simulink model "q_2dsfl_pos_cntrl"  (Simulink 7.0)
settings: Solver=ode1  StartTime=0.0  StopTime=inf  FixedStep=0.002  RelTol=1e-3
undefined symbols (not defined in the file or in its folder): DTH1_LIM_ENABLE, DTH2_LIM_ENABLE, DTH2_MAX, DTH2_MIN, HIL, K1, K1_defl_b, K1_strain_b, K2, K2_defl_b, K2_strain_b, KE_D1, KE_D2, LIMIT_SWITCHES_ENABLE, qc_get_step_size, wcf, wcfa, zetaf
libraries: quarc_library x21, simulink_extras x8, simulink x6
settings Model: Creator=ajavid  LastModifiedBy=MLevis  SimulationMode=external  ExtModeTrigDuration=60000
settings SolverCC: PositivePriorityOrder=on
settings DataIOCC: MaxDataPoints=30000
settings DebuggingCC: SaveWithParameterizedLinksMsg=none
settings RTWCC: SystemTargetFile=quarc_windows.tlc  TemplateMakefile=quarc_default_tmf  Description=QuaRC Win32 Target  ProcessScript=quarc_windows_make_rtw_hook
settings STFCustomTargetCC: TargetFcnLib=ansi_tfl_tmw.mat  TargetPreCompLibLocation=C:\DOCUME~1\ALLUSE~1\APPLIC~1\QUARC\lib\2007b\windows\release  GenFloatMathFcnCalls=ANSI_C  SystemTargetFile=quarc_windows.tlc
settings GRTTargetCC: TargetFcnLib=ansi_tfl_tmw.mat  TargetPreCompLibLocation=C:\DOCUME~1\ALLUSE~1\APPLIC~1\QUARC\lib\2007b\windows\release  CompOptLevelCompliant=off  MatFileLogging=off  ExtMode=on  ExtModeMexFile=quarc_comm

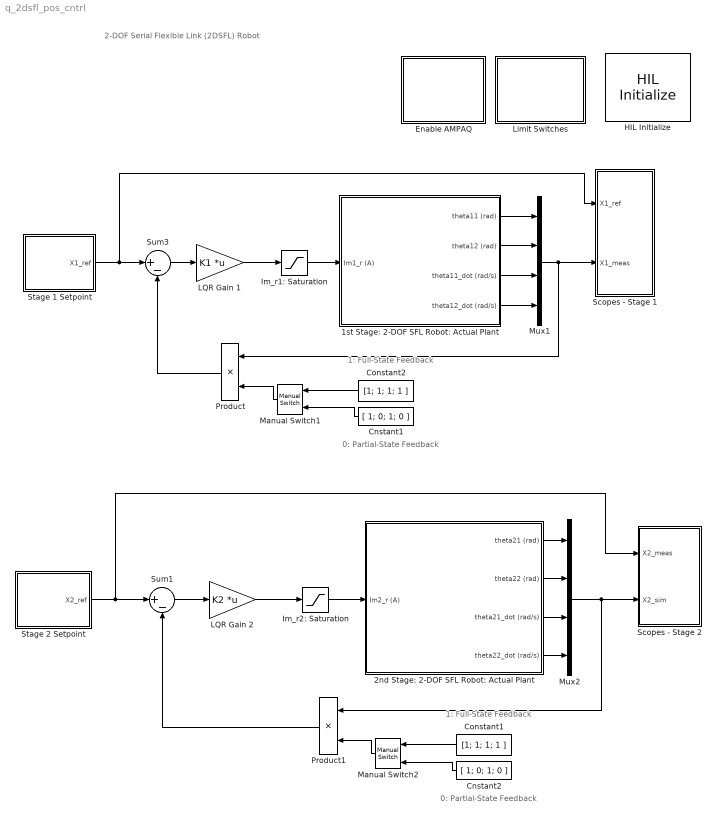
== system q_2dsfl_pos_cntrl ==
  note: 2-DOF Serial Flexible Link (2DSFL) Robot
  note: 1: Full-State Feedback
  note: 0: Partial-State Feedback
  note: 1: Full-State Feedback
  note: 0: Partial-State Feedback
  1st Stage: 2-DOF SFL Robot: Actual Plant : Subsystem
  2nd Stage: 2-DOF SFL Robot: Actual Plant : Subsystem
  Cnstant1 : Constant  Orientation=left  Value=[ 1; 0; 1; 0 ]  OutDataType=sfix(16)  OutScaling=2^0
  Cnstant2 : Constant  Orientation=left  Value=[ 1; 0; 1; 0 ]  OutDataType=sfix(16)  OutScaling=2^0
  Constant1 : Constant  Orientation=left  Value=[1; 1; 1; 1 ]  OutDataType=sfix(16)  OutScaling=2^0
  Constant2 : Constant  Orientation=left  Value=[1; 1; 1; 1 ]  OutDataType=sfix(16)  OutScaling=2^0
  Enable AMPAQ : Subsystem
  HIL Initialize : quarc_library/Data Acquisition/Generic/Configuration/HIL Initialize  object_name=HIL-1  board_type=q8  board_number=0  exclusive=off  active=on  hardware_clocks=[0:1]  clock_modes=[0 0]  initial_clock_frequencies=[]  set_clock_params_at_start=on  set_clock_params_at_switch_in=off  set_clock_frequencies_at_start=off  set_clock_frequencies_at_switch_in=off  analog_input_channels=[0:7]  analog_input_maximums=10  analog_input_minimums=-10  set_analog_input_params_at_start=off  set_analog_input_params_at_switch_in=off  analog_output_channels=[0:7]  analog_output_maximums=[10]  analog_output_minimums=[-10]  initial_analog_outputs=[0]  final_analog_outputs=[0]  watchdog_analog_outputs=0  set_analog_output_params_at_start=on  set_analog_output_params_at_switch_in=off  set_analog_outputs_at_start=on  set_analog_outputs_at_switch_in=off  set_analog_outputs_at_terminate=on  set_analog_outputs_at_switch_out=off  set_analog_outputs_on_watchdog=off  digital_input_channels=[8:31]  digital_output_channels=[0:7]  digital_output_configuration=[]  initial_digital_outputs=[1]  final_digital_outputs=[1]  watchdog_digital_outputs=[2]  set_digital_output_params_at_start=off  set_digital_output_params_at_switch_in=off  set_digital_outputs_at_start=on  set_digital_outputs_at_switch_in=off  set_digital_outputs_at_terminate=on  set_digital_outputs_at_switch_out=off  set_digital_outputs_on_watchdog=on  encoder_channels=[0:7]  quadrature=[4]  encoder_filter_frequency=(1/120e-9)/1  initial_encoder_counts=[0]  set_encoder_params_at_start=on  set_encoder_params_at_switch_in=off  set_encoder_counts_at_start=on  set_encoder_counts_at_switch_in=off  pwm_channels=[]  pwm_modes=[0]  pwm_frequency=(1/60e-9)/1024  pwm_configuration=[]  pwm_alignment=[]  pwm_polarity=[]  pwm_leading_deadband=[]  pwm_trailing_deadband=[]  initial_pwm_outputs=[0]  final_pwm_outputs=[0]  watchdog_pwm_outputs=[]  set_pwm_params_at_start=on  set_pwm_params_at_switch_in=off  set_pwm_outputs_at_start=on  set_pwm_outputs_at_switch_in=off  set_pwm_outputs_at_terminate=on  set_pwm_outputs_at_switch_out=off  set_pwm_outputs_on_watchdog=off  other_output_channels=[]  initial_other_outputs=[]  final_other_outputs=[]  watchdog_other_outputs=[]  set_other_outputs_at_start=off  set_other_outputs_at_switch_in=off  set_other_outputs_at_terminate=off  set_other_outputs_at_switch_out=off  set_other_outputs_on_watchdog=off
  Im_r1: Saturation : Saturate  UpperLimit=0.94  LowerLimit=-0.94
  Im_r2: Saturation : Saturate  UpperLimit=1.2  LowerLimit=-1.2
  LQR Gain 1 : Gain  Gain=K1  Multiplication=Matrix(K*u)  ParameterDataType=sfix(16)  ParameterScaling=2^0  OutDataType=sfix(16)  OutScaling=2^0
  LQR Gain 2 : Gain  Gain=K2  Multiplication=Matrix(K*u)  ParameterDataType=sfix(16)  ParameterScaling=2^0  OutDataType=sfix(16)  OutScaling=2^0
  Limit Switches : Subsystem
  Manual Switch1 : simulink/Signal Routing/Manual Switch  Orientation=left  SystemSampleTime=-1  sw=1  action=0  varsize=off
  Manual Switch2 : simulink/Signal Routing/Manual Switch  Orientation=left  SystemSampleTime=-1  sw=1  action=0  varsize=off
  Mux1 : Mux
  Mux2 : Mux
  Product : Product  Orientation=left  OutDataType=sfix(16)  OutScaling=2^0  SaturateOnIntegerOverflow=on  RndMeth=Zero  InputSameDT=on
  Product1 : Product  Orientation=left  OutDataType=sfix(16)  OutScaling=2^0  SaturateOnIntegerOverflow=on  RndMeth=Zero  InputSameDT=on
  Scopes - Stage 1 : Subsystem
  Scopes - Stage 2 : Subsystem
  Stage 1 Setpoint : Subsystem
  Stage 2 Setpoint : Subsystem
  Sum1 : Sum  Inputs=|+-  OutDataType=sfix(16)  OutScaling=2^0  SaturateOnIntegerOverflow=on  InputSameDT=on
  Sum3 : Sum  Inputs=|+-  OutDataType=sfix(16)  OutScaling=2^0  SaturateOnIntegerOverflow=on  InputSameDT=on
  wires:
  1st Stage: 2-DOF SFL Robot: Actual Plant/3(theta11_dot (rad/s)) -> Mux1/3
  1st Stage: 2-DOF SFL Robot: Actual Plant/4(theta12_dot (rad/s)) -> Mux1/4
  1st Stage: 2-DOF SFL Robot: Actual Plant/2(theta12 (rad)) -> Mux1/2
  1st Stage: 2-DOF SFL Robot: Actual Plant/1(theta11 (rad)) -> Mux1/1
  Mux1/1 -> Product/1, Scopes - Stage 1/2(X1_meas)
  2nd Stage: 2-DOF SFL Robot: Actual Plant/3(theta21_dot (rad/s)) -> Mux2/3
  2nd Stage: 2-DOF SFL Robot: Actual Plant/4(theta22_dot (rad/s)) -> Mux2/4
  2nd Stage: 2-DOF SFL Robot: Actual Plant/2(theta22 (rad)) -> Mux2/2
  2nd Stage: 2-DOF SFL Robot: Actual Plant/1(theta21 (rad)) -> Mux2/1
  Im_r2: Saturation/1 -> 2nd Stage: 2-DOF SFL Robot: Actual Plant/1(Im2_r (A))
  Constant2/1 -> Manual Switch1/1
  Cnstant1/1 -> Manual Switch1/2
  Manual Switch1/1 -> Product/2
  Im_r1: Saturation/1 -> 1st Stage: 2-DOF SFL Robot: Actual Plant/1(Im1_r (A))
  Stage 1 Setpoint/1(X1_ref) -> Sum3/1, Scopes - Stage 1/1(X1_ref)
  Sum3/1 -> LQR Gain 1/1
  Product/1 -> Sum3/2
  Stage 2 Setpoint/1(X2_ref) -> Sum1/1, Scopes - Stage 2/1(X2_meas)
  Sum1/1 -> LQR Gain 2/1
  LQR Gain 2/1 -> Im_r2: Saturation/1
  Mux2/1 -> Scopes - Stage 2/2(X2_sim), Product1/1
  LQR Gain 1/1 -> Im_r1: Saturation/1
  Constant1/1 -> Manual Switch2/1
  Cnstant2/1 -> Manual Switch2/2
  Manual Switch2/1 -> Product1/2
  Product1/1 -> Sum1/2

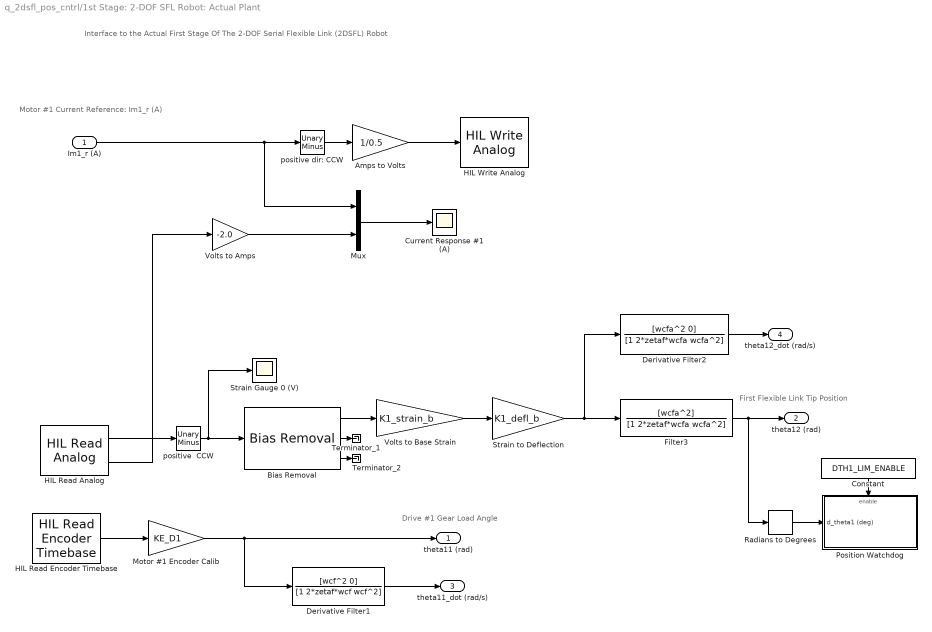
== system q_2dsfl_pos_cntrl/1st Stage: 2-DOF SFL Robot: Actual Plant ==
  note: Interface to the Actual
      | First Stage Of The 2-DOF Serial Flexible Link (2DSFL) Robot
  note: First Flexible Link
      | Tip Position
  note: Drive #1
      | Gear Load Angle
  note: Motor #1 Current Reference:
      | Im1_r (A)
  Im1_r (A) : Inport  OutDataType=sfix(16)  OutScaling=2^0
  Amps to Volts : Gain  Gain=1/0.5  ParameterDataType=sfix(16)  ParameterScaling=2^0  OutDataType=sfix(16)  OutScaling=2^0  SaturateOnIntegerOverflow=on
  Bias Removal : quarc_library/Discrete/Bias Removal  SystemSampleTime=-1  start_time=0  end_time=1  switch_id=0  sample_time=qc_get_step_size
  Constant : Constant  Orientation=down  Value=DTH1_LIM_ENABLE  OutDataType=sfix(16)  OutScaling=2^0
  Current Response #1 (A) : Scope
      settings: TimeRange=20  YMin=-1  YMax=1  SaveName=data_Im1  DataFormat=Array  MaxDataPoints=10000
  Derivative Filter1 : TransferFcn  Numerator=[wcf^2 0]  Denominator=[1 2*zetaf*wcf wcf^2]
  Derivative Filter2 : TransferFcn  Numerator=[wcfa^2 0]  Denominator=[1 2*zetaf*wcfa wcfa^2]
  Filter3 : TransferFcn  Numerator=[wcfa^2]  Denominator=[1 2*zetaf*wcfa wcfa^2]
  HIL Read Analog : quarc_library/Data Acquisition/Generic/Immediate I//O/HIL Read Analog  object_name=HIL-1  channels=[0,2]  sample_time=qc_get_step_size  active=on  vector_output=off
  HIL Read Encoder Timebase : quarc_library/Data Acquisition/Generic/Timebases/HIL Read Encoder Timebase  object_name=HIL-1  clock=0  channels=0  samples_in_buffer=max(ceil(1/qc_get_step_size), 1)  active=on  vector_output=off  data_type_mode=Inherit via back propagation  data_type=double
  HIL Write Analog : quarc_library/Data Acquisition/Generic/Immediate I//O/HIL Write Analog  object_name=HIL-1  channels=0  sample_time=-1  active=off  vector_input=off
  Motor #1 Encoder Calib : Gain  Gain=KE_D1  ParameterDataType=sfix(16)  ParameterScaling=2^0  OutDataType=sfix(16)  OutScaling=2^0  SaturateOnIntegerOverflow=on
  Mux : Mux  Inputs=2
  Position Watchdog : Subsystem  TreatAsAtomicUnit=on
  Radians to Degrees : simulink_extras/Transformations/Radians to Degrees  SystemSampleTime=-1
  Strain Gauge 0 (V) : Scope
      settings: TickLabels=on  TimeRange=2  YMin=-1.5  YMax=1.5  SaveName=ScopeData7  DataFormat=Array
  Strain to Deflection : Gain  Gain=K1_defl_b  ParameterDataType=sfix(16)  ParameterScaling=2^0  OutDataType=sfix(16)  OutScaling=2^0  SaturateOnIntegerOverflow=on
  Terminator_1 : Terminator
  Terminator_2 : Terminator
  Volts to Amps : Gain  Gain=-2.0  ParameterDataType=sfix(16)  ParameterScaling=2^0  OutDataType=sfix(16)  OutScaling=2^0
  Volts to Base Strain : Gain  Gain=K1_strain_b  ParameterDataType=sfix(16)  ParameterScaling=2^0  OutDataType=sfix(16)  OutScaling=2^0  SaturateOnIntegerOverflow=on
  positive  CCW : simulink/Math Operations/Unary Minus  DoSatur=off
  positive dir: CCW : simulink/Math Operations/Unary Minus  DoSatur=off
  theta11 (rad) : Outport  OutDataType=sfix(16)  OutScaling=2^0  InitialOutput=0
  theta12 (rad) : Outport  Port=2  OutDataType=sfix(16)  OutScaling=2^0  InitialOutput=0
  theta11_dot (rad/s) : Outport  Port=3  OutDataType=sfix(16)  OutScaling=2^0  InitialOutput=0
  theta12_dot (rad/s) : Outport  Port=4  OutDataType=sfix(16)  OutScaling=2^0  InitialOutput=0
  wires:
  positive  CCW/1 -> Strain Gauge 0 (V)/1, Bias Removal/1
  Filter3/1 -> theta12 (rad)/1, Radians to Degrees/1
  Derivative Filter1/1 -> theta11_dot (rad/s)/1
  Derivative Filter2/1 -> theta12_dot (rad/s)/1
  Strain to Deflection/1 -> Filter3/1, Derivative Filter2/1
  Im1_r (A)/1 -> positive dir: CCW/1, Mux/1
  HIL Read Encoder Timebase/1 -> Motor #1 Encoder Calib/1
  Volts to Amps/1 -> Mux/2
  Mux/1 -> Current Response #1 (A)/1
  Motor #1 Encoder Calib/1 -> Derivative Filter1/1, theta11 (rad)/1
  HIL Read Analog/1 -> positive  CCW/1
  positive dir: CCW/1 -> Amps to Volts/1
  Volts to Base Strain/1 -> Strain to Deflection/1
  Amps to Volts/1 -> HIL Write Analog/1
  HIL Read Analog/2 -> Volts to Amps/1
  Constant/1 -> Position Watchdog/Enable
  Radians to Degrees/1 -> Position Watchdog/1(d_theta1 (deg))
  Bias Removal/1 -> Volts to Base Strain/1
  Bias Removal/2 -> Terminator_1/1
  Bias Removal/3 -> Terminator_2/1

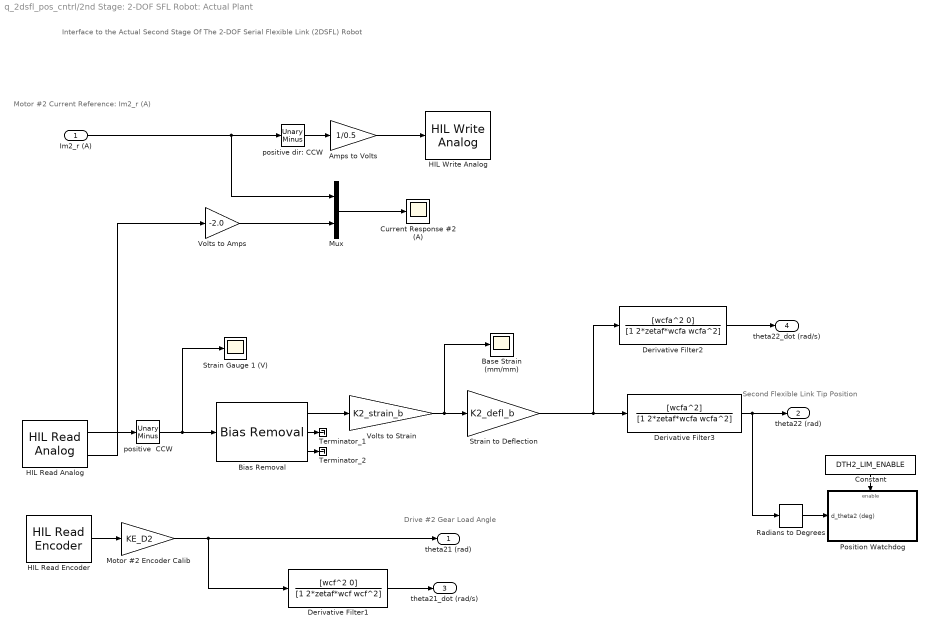
== system q_2dsfl_pos_cntrl/2nd Stage: 2-DOF SFL Robot: Actual Plant ==
  note: Motor #2 Current Reference:
      | Im2_r (A)
  note: Drive #2
      | Gear Load Angle
  note: Second Flexible Link
      | Tip Position
  note: Interface to the Actual
      | Second Stage Of The 2-DOF Serial Flexible Link (2DSFL) Robot
  Im2_r (A) : Inport  OutDataType=sfix(16)  OutScaling=2^0
  Amps to Volts : Gain  Gain=1/0.5  ParameterDataType=sfix(16)  ParameterScaling=2^0  OutDataType=sfix(16)  OutScaling=2^0  SaturateOnIntegerOverflow=on
  Base Strain (mm/mm) : Scope
      settings: TickLabels=on  TimeRange=1.000000  YMin=-1  YMax=1  SaveName=ScopeData4  DataFormat=Array
  Bias Removal : quarc_library/Discrete/Bias Removal  SystemSampleTime=-1  start_time=0  end_time=0.2  switch_id=0  sample_time=qc_get_step_size
  Constant : Constant  Orientation=down  Value=DTH2_LIM_ENABLE  OutDataType=sfix(16)  OutScaling=2^0
  Current Response #2 (A) : Scope
      settings: TimeRange=20  YMin=-1.25  YMax=1.25  SaveName=data_Im2  DataFormat=Array  MaxDataPoints=10000
  Derivative Filter1 : TransferFcn  Numerator=[wcf^2 0]  Denominator=[1 2*zetaf*wcf wcf^2]
  Derivative Filter2 : TransferFcn  Numerator=[wcfa^2 0]  Denominator=[1 2*zetaf*wcfa wcfa^2]
  Derivative Filter3 : TransferFcn  Numerator=[wcfa^2]  Denominator=[1 2*zetaf*wcfa wcfa^2]
  HIL Read Analog : quarc_library/Data Acquisition/Generic/Immediate I//O/HIL Read Analog  object_name=HIL-1  channels=[1,3]  sample_time=qc_get_step_size  active=on  vector_output=off
  HIL Read Encoder : quarc_library/Data Acquisition/Generic/Immediate I//O/HIL Read Encoder  object_name=HIL-1  channels=1  sample_time=qc_get_step_size  active=on  vector_output=off  data_type_mode=Inherit via back propagation  data_type=double
  HIL Write Analog : quarc_library/Data Acquisition/Generic/Immediate I//O/HIL Write Analog  object_name=HIL-1  channels=1  sample_time=-1  active=off  vector_input=off
  Motor #2 Encoder Calib : Gain  Gain=KE_D2  ParameterDataType=sfix(16)  ParameterScaling=2^0  OutDataType=sfix(16)  OutScaling=2^0  SaturateOnIntegerOverflow=on
  Mux : Mux  Inputs=2
  Position Watchdog : Subsystem  TreatAsAtomicUnit=on
  Radians to Degrees : simulink_extras/Transformations/Radians to Degrees  SystemSampleTime=-1
  Strain Gauge 1 (V) : Scope
      settings: TickLabels=on  TimeRange=1.000000  YMin=-1  YMax=1  SaveName=ScopeData7  DataFormat=Array
  Strain to Deflection : Gain  Gain=K2_defl_b  ParameterDataType=sfix(16)  ParameterScaling=2^0  OutDataType=sfix(16)  OutScaling=2^0  SaturateOnIntegerOverflow=on
  Terminator_1 : Terminator
  Terminator_2 : Terminator
  Volts to Amps : Gain  Gain=-2.0  ParameterDataType=sfix(16)  ParameterScaling=2^0  OutDataType=sfix(16)  OutScaling=2^0
  Volts to Strain : Gain  Gain=K2_strain_b  ParameterDataType=sfix(16)  ParameterScaling=2^0  OutDataType=sfix(16)  OutScaling=2^0  SaturateOnIntegerOverflow=on
  positive  CCW : simulink/Math Operations/Unary Minus  DoSatur=off
  positive dir: CCW : simulink/Math Operations/Unary Minus  DoSatur=off
  theta21 (rad) : Outport  OutDataType=sfix(16)  OutScaling=2^0  InitialOutput=0
  theta22 (rad) : Outport  Port=2  OutDataType=sfix(16)  OutScaling=2^0  InitialOutput=0
  theta21_dot (rad/s) : Outport  Port=3  OutDataType=sfix(16)  OutScaling=2^0  InitialOutput=0
  theta22_dot (rad/s) : Outport  Port=4  OutDataType=sfix(16)  OutScaling=2^0  InitialOutput=0
  wires:
  Derivative Filter3/1 -> theta22 (rad)/1, Radians to Degrees/1
  positive  CCW/1 -> Strain Gauge 1 (V)/1, Bias Removal/1
  Derivative Filter2/1 -> theta22_dot (rad/s)/1
  Strain to Deflection/1 -> Derivative Filter3/1, Derivative Filter2/1
  Derivative Filter1/1 -> theta21_dot (rad/s)/1
  Volts to Strain/1 -> Strain to Deflection/1, Base Strain (mm/mm)/1
  HIL Read Analog/1 -> positive  CCW/1
  HIL Read Analog/2 -> Volts to Amps/1
  Mux/1 -> Current Response #2 (A)/1
  Volts to Amps/1 -> Mux/2
  HIL Read Encoder/1 -> Motor #2 Encoder Calib/1
  Motor #2 Encoder Calib/1 -> theta21 (rad)/1, Derivative Filter1/1
  Im2_r (A)/1 -> positive dir: CCW/1, Mux/1
  Amps to Volts/1 -> HIL Write Analog/1
  Bias Removal/1 -> Volts to Strain/1
  Constant/1 -> Position Watchdog/Enable
  Radians to Degrees/1 -> Position Watchdog/1(d_theta2 (deg))
  Bias Removal/2 -> Terminator_1/1
  positive dir: CCW/1 -> Amps to Volts/1
  Bias Removal/3 -> Terminator_2/1

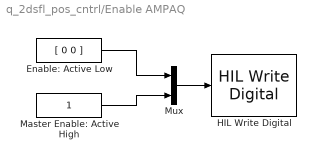
== system q_2dsfl_pos_cntrl/Enable AMPAQ ==
  Enable: Active Low : Constant  Value=[ 0 0 ]  OutDataType=sfix(16)  OutScaling=2^0
  HIL Write Digital : quarc_library/Data Acquisition/Generic/Immediate I//O/HIL Write Digital  object_name=HIL-1  channels=[0 1 4]  sample_time=-1  active=off  vector_input=on
  Master Enable: Active High : Constant  OutDataType=sfix(16)  OutScaling=2^0
  Mux : Mux  Inputs=2
  wires:
  Master Enable: Active High/1 -> Mux/2
  Enable: Active Low/1 -> Mux/1
  Mux/1 -> HIL Write Digital/1

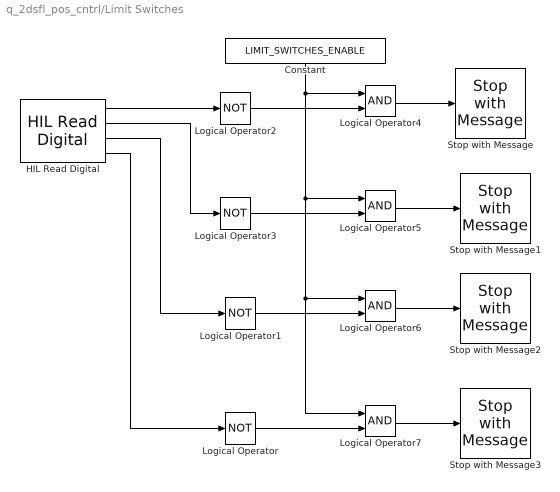
== system q_2dsfl_pos_cntrl/Limit Switches ==
  Constant : Constant  Orientation=down  Value=LIMIT_SWITCHES_ENABLE  OutDataType=sfix(16)  OutScaling=2^0
  HIL Read Digital : quarc_library/Data Acquisition/Generic/Immediate I//O/HIL Read Digital  object_name=HIL-1  channels=[8:11]  sample_time=qc_get_step_size  active=on  vector_output=off  data_type_mode=Inherit via back propagation  data_type=boolean
      settings: AttributesFormatString=(%<object_name>)
  Logical Operator{,1..3} (4 alike) : Logic  Operator=NOT  AllPortsSameDT=off  OutDataTypeMode=boolean
  Logical Operator{4..7} (4 alike) : Logic  AllPortsSameDT=off  OutDataTypeMode=boolean
  Stop with Message : quarc_library/Sinks/Error Handling/Stop with Message  SystemSampleTime=-1  message_type=Fixed error message  message_icon=Error  message=STAGE 1: MAX limit switch hit.
  Stop with Message1 : quarc_library/Sinks/Error Handling/Stop with Message  SystemSampleTime=-1  message_type=Fixed error message  message_icon=Error  message=STAGE 1: MIN limit switch hit.
  Stop with Message2 : quarc_library/Sinks/Error Handling/Stop with Message  SystemSampleTime=-1  message_type=Fixed error message  message_icon=Error  message=STAGE 2: MAX limit switch hit.
  Stop with Message3 : quarc_library/Sinks/Error Handling/Stop with Message  SystemSampleTime=-1  message_type=Fixed error message  message_icon=Error  message=STAGE 2: MIN limit switch hit.
  wires:
  Logical Operator7/1 -> Stop with Message3/1
  Logical Operator6/1 -> Stop with Message2/1
  Logical Operator5/1 -> Stop with Message1/1
  Logical Operator4/1 -> Stop with Message/1
  HIL Read Digital/4 -> Logical Operator/1
  HIL Read Digital/3 -> Logical Operator1/1
  HIL Read Digital/2 -> Logical Operator3/1
  HIL Read Digital/1 -> Logical Operator2/1
  Logical Operator2/1 -> Logical Operator4/2
  Constant/1 -> Logical Operator4/1, Logical Operator5/1, Logical Operator6/1, Logical Operator7/1
  Logical Operator3/1 -> Logical Operator5/2
  Logical Operator1/1 -> Logical Operator6/2
  Logical Operator/1 -> Logical Operator7/2

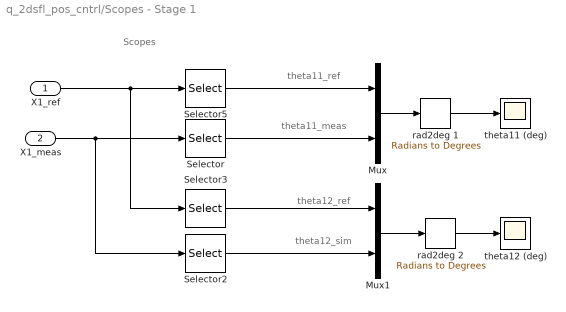
== system q_2dsfl_pos_cntrl/Scopes - Stage 1 ==
  note: Scopes
  note: theta12_sim
  note: theta11_ref
  note: theta11_meas
  note: theta12_ref
  X1_ref : Inport  OutDataType=sfix(16)  OutScaling=2^0
  X1_meas : Inport  Port=2  OutDataType=sfix(16)  OutScaling=2^0
  Mux : Mux  Inputs=2
  Mux1 : Mux  Inputs=2
  Selector : Selector  InputPortWidth=4  IndexOptions=Index vector (dialog)  Indices=[1]  OutputSizes=1
  Selector2 : Selector  InputPortWidth=4  IndexOptions=Index vector (dialog)  Indices=[2]  OutputSizes=1
  Selector3 : Selector  InputPortWidth=4  IndexOptions=Index vector (dialog)  Indices=[2]  OutputSizes=1
  Selector5 : Selector  InputPortWidth=4  IndexOptions=Index vector (dialog)  Indices=[1]  OutputSizes=1
  rad2deg 1 : simulink_extras/Transformations/Radians to Degrees  SystemSampleTime=-1
  rad2deg 2 : simulink_extras/Transformations/Radians to Degrees  SystemSampleTime=-1
  theta11 (deg) : Scope
      settings: TickLabels=on  TimeRange=20  YMin=-30  YMax=30  SaveName=data_th11  DataFormat=Array  MaxDataPoints=10000
  theta12 (deg) : Scope
      settings: TimeRange=20  YMin=-2  YMax=2  SaveName=data_th12  DataFormat=Array  MaxDataPoints=10000
  wires:
  X1_ref/1 -> Selector3/1, Selector5/1
  Mux/1 -> rad2deg 1/1
  Mux1/1 -> rad2deg 2/1
  X1_meas/1 -> Selector/1, Selector2/1
  rad2deg 1/1 -> theta11 (deg)/1
  rad2deg 2/1 -> theta12 (deg)/1
  Selector5/1 -> Mux/1
  Selector/1 -> Mux/2
  Selector2/1 -> Mux1/2
  Selector3/1 -> Mux1/1

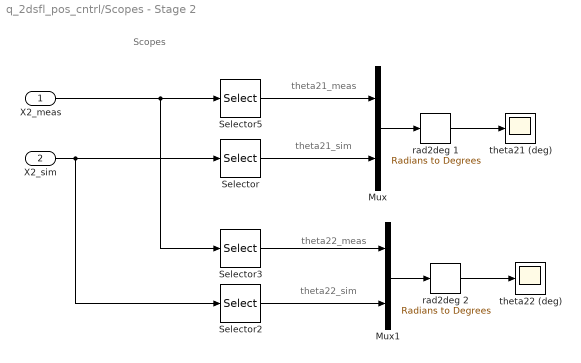
== system q_2dsfl_pos_cntrl/Scopes - Stage 2 ==
  note: Scopes
  note: theta22_sim
  note: theta21_sim
  note: theta21_meas
  note: theta22_meas
  X2_meas : Inport  OutDataType=sfix(16)  OutScaling=2^0
  X2_sim : Inport  Port=2  OutDataType=sfix(16)  OutScaling=2^0
  Mux : Mux  Inputs=2
  Mux1 : Mux  Inputs=2
  Selector : Selector  InputPortWidth=4  IndexOptions=Index vector (dialog)  Indices=[1]  OutputSizes=1
  Selector2 : Selector  InputPortWidth=4  IndexOptions=Index vector (dialog)  Indices=[2]  OutputSizes=1
  Selector3 : Selector  InputPortWidth=4  IndexOptions=Index vector (dialog)  Indices=[2]  OutputSizes=1
  Selector5 : Selector  InputPortWidth=4  IndexOptions=Index vector (dialog)  Indices=[1]  OutputSizes=1
  rad2deg 1 : simulink_extras/Transformations/Radians to Degrees  SystemSampleTime=-1
  rad2deg 2 : simulink_extras/Transformations/Radians to Degrees  SystemSampleTime=-1
  theta21 (deg) : Scope
      settings: TickLabels=on  TimeRange=20  YMin=-15  YMax=15  SaveName=data_th21  DataFormat=Array  MaxDataPoints=10000
  theta22 (deg) : Scope
      settings: TimeRange=20  YMin=-2.5  YMax=2.5  SaveName=data_th22  DataFormat=Array  MaxDataPoints=10000
  wires:
  Mux/1 -> rad2deg 1/1
  Mux1/1 -> rad2deg 2/1
  X2_meas/1 -> Selector3/1, Selector5/1
  X2_sim/1 -> Selector2/1, Selector/1
  rad2deg 1/1 -> theta21 (deg)/1
  rad2deg 2/1 -> theta22 (deg)/1
  Selector3/1 -> Mux1/1
  Selector2/1 -> Mux1/2
  Selector5/1 -> Mux/1
  Selector/1 -> Mux/2

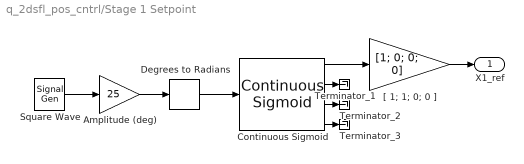
== system q_2dsfl_pos_cntrl/Stage 1 Setpoint ==
  Amplitude (deg) : Gain  Gain=25  ParameterDataType=sfix(16)  ParameterScaling=2^0  OutDataType=sfix(16)  OutScaling=2^0  SaturateOnIntegerOverflow=on
  Continuous Sigmoid : quarc_library/Sources/Sigmoids/Continuous Sigmoid  params_source=Internal (dialog parameters)  max_velocity=2.35  max_acceleration=4.45  initial_position=0  initial_velocity=0  hold_off=0.5  input_sample_time=-1  output_sample_time=qc_get_step_size
  Degrees to Radians : simulink_extras/Transformations/Degrees to Radians  SystemSampleTime=-1
  Square Wave : SignalGenerator  WaveForm=square  Frequency=0.1
  Terminator_1 : Terminator
  Terminator_2 : Terminator
  Terminator_3 : Terminator
  "[ 1; 1; 0; 0 ]" : Gain  Gain=[1; 0; 0; 0]  ParameterDataType=sfix(16)  ParameterScaling=2^0  OutDataType=sfix(16)  OutScaling=2^0  SaturateOnIntegerOverflow=on
  X1_ref : Outport
  wires:
  Continuous Sigmoid/1 -> "[ 1; 1; 0; 0 ]"/1
  Continuous Sigmoid/4 -> Terminator_3/1
  Continuous Sigmoid/3 -> Terminator_2/1
  Continuous Sigmoid/2 -> Terminator_1/1
  Degrees to Radians/1 -> Continuous Sigmoid/1
  "[ 1; 1; 0; 0 ]"/1 -> X1_ref/1
  Amplitude (deg)/1 -> Degrees to Radians/1
  Square Wave/1 -> Amplitude (deg)/1

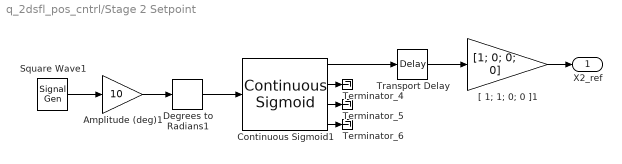
== system q_2dsfl_pos_cntrl/Stage 2 Setpoint ==
  Amplitude (deg)1 : Gain  Gain=10  ParameterDataType=sfix(16)  ParameterScaling=2^0  OutDataType=sfix(16)  OutScaling=2^0  SaturateOnIntegerOverflow=on
  Continuous Sigmoid1 : quarc_library/Sources/Sigmoids/Continuous Sigmoid  params_source=Internal (dialog parameters)  max_velocity=2  max_acceleration=5  initial_position=0  initial_velocity=0  hold_off=0.5  input_sample_time=-1  output_sample_time=qc_get_step_size
  Degrees to Radians1 : simulink_extras/Transformations/Degrees to Radians  SystemSampleTime=-1
  Square Wave1 : SignalGenerator  WaveForm=square  Frequency=0.1
  Terminator_4 : Terminator
  Terminator_5 : Terminator
  Terminator_6 : Terminator
  Transport Delay : TransportDelay  DelayTime=2.5  BufferSize=10/qc_get_step_size
  "[ 1; 1; 0; 0 ]1" : Gain  Gain=[1; 0; 0; 0]  ParameterDataType=sfix(16)  ParameterScaling=2^0  OutDataType=sfix(16)  OutScaling=2^0  SaturateOnIntegerOverflow=on
  X2_ref : Outport
  wires:
  "[ 1; 1; 0; 0 ]1"/1 -> X2_ref/1
  Degrees to Radians1/1 -> Continuous Sigmoid1/1
  Continuous Sigmoid1/4 -> Terminator_6/1
  Continuous Sigmoid1/3 -> Terminator_5/1
  Continuous Sigmoid1/2 -> Terminator_4/1
  Amplitude (deg)1/1 -> Degrees to Radians1/1
  Square Wave1/1 -> Amplitude (deg)1/1
  Transport Delay/1 -> "[ 1; 1; 0; 0 ]1"/1
  Continuous Sigmoid1/1 -> Transport Delay/1

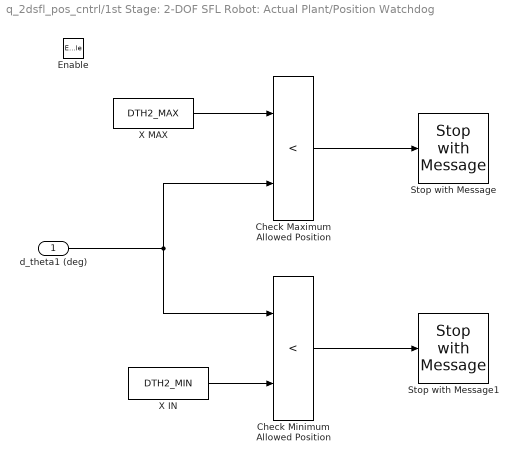
== system q_2dsfl_pos_cntrl/1st Stage: 2-DOF SFL Robot: Actual Plant/Position Watchdog ==
  d_theta1 (deg) : Inport  OutDataType=sfix(16)  OutScaling=2^0
  Enable : EnablePort
  Check Maximum Allowed Position : RelationalOperator  Operator=<  InputSameDT=on
  Check Minimum Allowed Position : RelationalOperator  Operator=<  InputSameDT=on
  Stop with Message : quarc_library/Sinks/Error Handling/Stop with Message  SystemSampleTime=-1  message_type=Fixed error message  message_icon=Error  message=Stage 1 link went above DTH1_MAX variable.
  Stop with Message1 : quarc_library/Sinks/Error Handling/Stop with Message  SystemSampleTime=-1  message_type=Fixed error message  message_icon=Error  message=Stage 1 link went below DTH1_MIN variable.
  X IN : Constant  Value=DTH2_MIN  OutDataType=sfix(16)  OutScaling=2^0
  X MAX : Constant  Value=DTH2_MAX  OutDataType=sfix(16)  OutScaling=2^0
  wires:
  d_theta1 (deg)/1 -> Check Minimum Allowed Position/1, Check Maximum Allowed Position/2
  X IN/1 -> Check Minimum Allowed Position/2
  X MAX/1 -> Check Maximum Allowed Position/1
  Check Maximum Allowed Position/1 -> Stop with Message/1
  Check Minimum Allowed Position/1 -> Stop with Message1/1

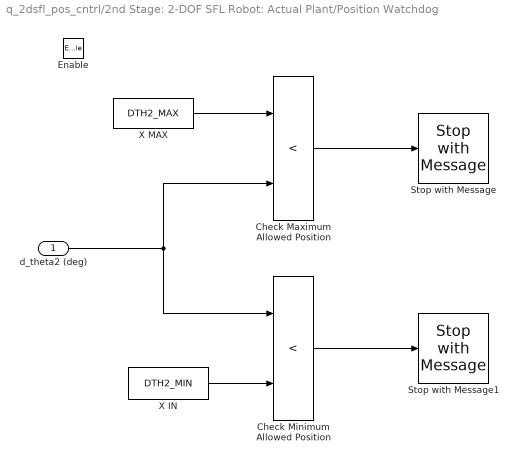
== system q_2dsfl_pos_cntrl/2nd Stage: 2-DOF SFL Robot: Actual Plant/Position Watchdog ==
  d_theta2 (deg) : Inport  OutDataType=sfix(16)  OutScaling=2^0
  Enable : EnablePort
  Check Maximum Allowed Position : RelationalOperator  Operator=<  InputSameDT=on
  Check Minimum Allowed Position : RelationalOperator  Operator=<  InputSameDT=on
  Stop with Message : quarc_library/Sinks/Error Handling/Stop with Message  SystemSampleTime=-1  message_type=Fixed error message  message_icon=Error  message=Stage 2 link went above DTH2_MAX variable.
  Stop with Message1 : quarc_library/Sinks/Error Handling/Stop with Message  SystemSampleTime=-1  message_type=Fixed error message  message_icon=Error  message=Stage 2 link went below DTH2_MIN variable.
  X IN : Constant  Value=DTH2_MIN  OutDataType=sfix(16)  OutScaling=2^0
  X MAX : Constant  Value=DTH2_MAX  OutDataType=sfix(16)  OutScaling=2^0
  wires:
  d_theta2 (deg)/1 -> Check Minimum Allowed Position/1, Check Maximum Allowed Position/2
  X IN/1 -> Check Minimum Allowed Position/2
  X MAX/1 -> Check Maximum Allowed Position/1
  Check Maximum Allowed Position/1 -> Stop with Message/1
  Check Minimum Allowed Position/1 -> Stop with Message1/1
